simulink model "V2G_FDCC"  (R2024a)
settings: Solver=FixedStepAuto  StartTime=0.0  StopTime=20  FixedStep=1e-5  MaxStep=1.0E-5  RelTol=1e-3
values from neighbouring files (symbols this model uses):
  C_inv = (r*(Pinv/3)*al*(-be+al-1))/(100*Vac_l_rms*Vin_inv*wn*(al-be))    [main_v2gg2v.m]
  C_mppt = 20*(Iout_mppt*D_mppt)/(deltaV*fs_mppt)    (= 0.0948148148148)    [main_v2gg2v.m]
  cap_bat = 2000    [main_v2gg2v.m]
  Cbat_buck = deltaI_bat/(8*fs_bat*deltaV_bat)    (= 0.00133333333333)    [main_v2gg2v.m]
  Cdc = 30e-3    (= 0.03)    [main_v2gg2v.m]
  Cdc_boost = 50*Cbat_buck    (= 0.0666666666667)    [main_v2gg2v.m]
  D = 5    [main_v2gg2v.m]    (also in test.m = [0; 1; 4; 8; 1; 10; 0.5; 0.1; 0.5; 2; 4; 12; 1; 1; 1; 1])
  Dinv = results.Dinv(comb_idx)    [calculate_cct.m]    (also in main_v2gg2v.m = 7)
  f_grid = 50    [main_v2gg2v.m]
  fg = 50    [main_v2gg2v.m]
  H1 = 3    [main_v2gg2v.m]
  H2 = 4    [main_v2gg2v.m]
  H3 = 5    [main_v2gg2v.m]
  Hinv = results.Hinv(comb_idx)    [calculate_cct.m]    (also in main_v2gg2v.m = 3)
  L_bat = (Vbat*(Vdc_link-Vbat))/(deltaI_bat*fs_bat*Vdc_link)    (= 0.001875)    [main_v2gg2v.m]
  L_mppt = 1*(Vpv*D_mppt)/(deltaI*fs_mppt)    (= 0.000161333333333)    [main_v2gg2v.m]
  Lmin_inv = (100*Vac_l_rms*Vin_inv*(al-be))/(wn*r*(Pinv/3)*(-be+al-1))    [main_v2gg2v.m]
  Pinv = 2e6    (= 2000000)    [main_v2gg2v.m]
  Sbase = 1e6    (= 1000000)    [main_v2gg2v.m]
  t_fault_end = t_fault_start + FCT    [calculate_cct.m]    (also in main_v2gg2v.m = 1.02)
  t_fault_start = 1    [calculate_cct.m]    (also in main_v2gg2v.m)
  Vac_inv = 800    [main_v2gg2v.m]
  Vbase = 345e3    (= 345000)    [main_v2gg2v.m]
  Vbat = 750    [main_v2gg2v.m]
  wg = 2*pi*fg    (= 314.159265359)    [main_v2gg2v.m]
undefined symbols (not defined in the file or in its folder): Acid, D1, Delta, L12, L13, L23, Lead
libraries: spsGroundLib x48, spsSeriesRLCBranchLib x32, eeGeneralControl x27, slpidlib x24, spsCurrentMeasurementLib x18, spsThreePhaseSeriesRLCBranchLib x15, spsThreePhaseVIMeasurementLib x14, spsVoltageMeasurementLib x11, spsBatteryLib x10, spsMosfetLib x8, spsPWMGeneratorDCDCLib x8, spsabctodq0Lib x8
(part 1 of 4)
settings Model: SimulationMode=accelerator  Creator=BagaskaraPP  LastModifiedBy=hp
settings SolverCC: ZeroCrossAlgorithm=Adaptive  AlgebraicLoopSolver=TrustRegion
settings DataIOCC: ExternalInput=getinputstruct(op1)  InitialState=getstatestruct(op1)  SaveFinalState=on  SaveOperatingPoint=on  SaveFormat=Structure  ReturnWorkspaceOutputs=off  Refine=4
settings DebuggingCC: AlgebraicLoopMsg=none  MaxConsecutiveZCsMsg=none  IgnoredZcDiagnostic=none  ArithmeticOperatorsInVariantConditions=warning
settings ModelReferenceCC: EnableRefExpFcnMdlSchedulingChecks=on
settings SFSimCC: SimUseLocalCustomCode=off  CustomCodeUndefinedFunction=UseInterfaceOnly
settings RTWCC: RTWUseLocalCustomCode=off  GPUComputeCapability=3.5
settings CodeAppCC: StateflowObjectComments=on
settings SimscapeCC: SimscapeNormalizeSystem=off

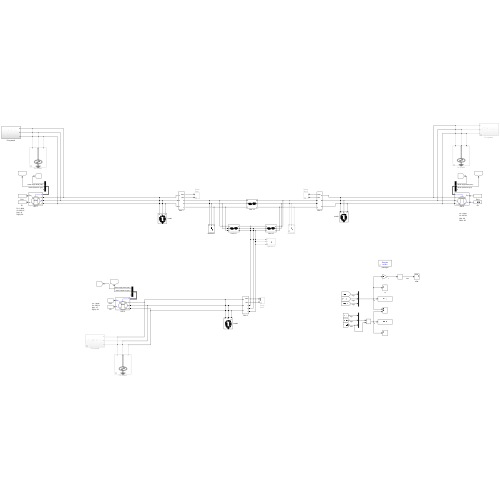
[thumbnail: Simulink's stored preview of the top-level diagram]
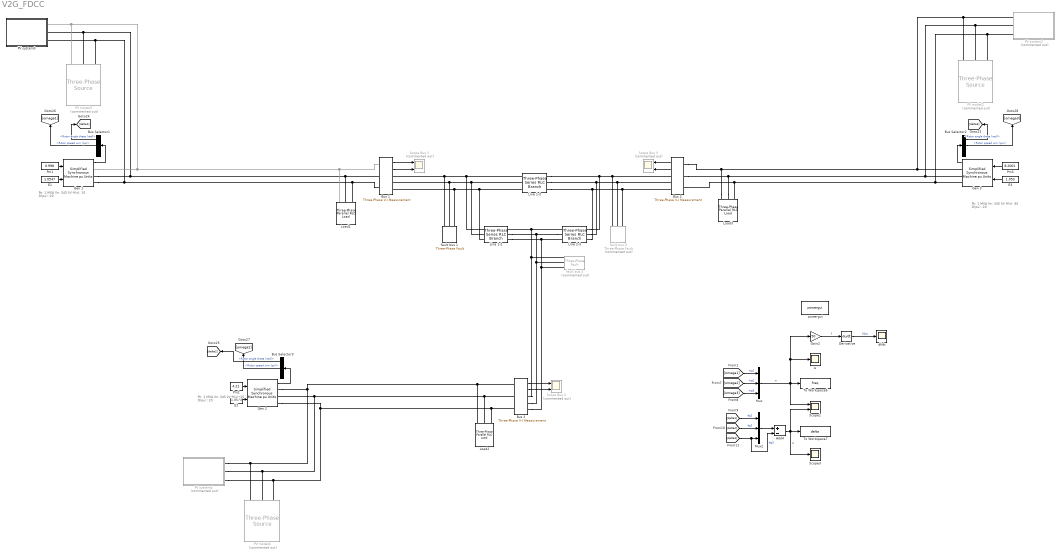
== system V2G_FDCC ==
  note: Pn: 1 MVA
      | Vn: 345 kV
      | H(s): 15
      | D(pu): 20
  note: Pn: 1 MVA
      | Vn: 345 kV
      | H(s): 60
      | D(pu): 20
  note: Pn: 1 MVA
      | Vn: 345 kV
      | H(s): 10
      | D(pu): 20
  Add4 : Sum  Inputs=+-
  Bus Selector1 : BusSelector  OutputSignals=Rotor angle theta (rad),Rotor speed wm (pu),Electrical power Pe (pu)
  Bus Selector2 : BusSelector  OutputSignals=Rotor angle theta (rad),Rotor speed wm (pu),Electrical power Pe (pu)
  Bus Selector3 : BusSelector  OutputSignals=Rotor angle theta (rad),Rotor speed wm (pu),Electrical power Pe (pu)
  Bus 1 : spsThreePhaseVIMeasurementLib/Three-Phase V-I Measurement  VoltageMeasurement=phase-to-ground  SetLabelV=off  LabelV=Vabc  Vpu=off  VpuLL=off  CurrentMeasurement=yes  SetLabelI=off  LabelI=Iabc  Ipu=off  Pbase=100e6  Vbase=500e3  OutputType=Complex  PhasorSimulation=off  PSBequivalent=0
  Bus 2 : spsThreePhaseVIMeasurementLib/Three-Phase V-I Measurement  VoltageMeasurement=phase-to-ground  SetLabelV=off  LabelV=Vabc  Vpu=off  VpuLL=off  CurrentMeasurement=yes  SetLabelI=off  LabelI=Iabc  Ipu=off  Pbase=100e6  Vbase=500e3  OutputType=Complex  PhasorSimulation=off  PSBequivalent=0
  Bus 3 : spsThreePhaseVIMeasurementLib/Three-Phase V-I Measurement  VoltageMeasurement=phase-to-ground  SetLabelV=off  LabelV=Vabc  Vpu=off  VpuLL=off  CurrentMeasurement=yes  SetLabelI=off  LabelI=Iabc  Ipu=off  Pbase=100e6  Vbase=500e3  OutputType=Complex  PhasorSimulation=off  PSBequivalent=0
  Derivative : Derivative
  E1 : Constant  Value=1.0547
  E2 : Constant  Value=1.0573
  E3 : Constant  Value=1.053
  Gain2 : Gain  Gain=50
  Gen 1 : spsSimplifiedSynchronousMachinepuUnitsLib/Simplified Synchronous Machine pu Units  ConnectionType=3-wire Y  MechanicalLoad=Mechanical power Pm  MeasurementBus=off  NominalParameters=[Sbase Vbase f_grid]  Mechanical=[H1 D 1]  InternalRL="[0.0  0.088]"  InitialConditions=[0 19.7182 1.15402 1.15402 1.15402 -15.1984 -135.198 104.802]  IterativeDiscreteModel=Trapezoidal non iterative  TsBlock=-1  TsPowergui=0  LoadFlowParameters=[1,0,0,0,0]  Units=0  BusType=PV  Pref=998000  Qref=0  Qmin=-Inf  Qmax=Inf  PLF=0  QLF=0
      settings: LibrarySourceBlock=|
      | sps_lib/Electrical Machines/Simplified Synchronous
      | Machine pu Units
  Gen 2 : spsSimplifiedSynchronousMachinepuUnitsLib/Simplified Synchronous Machine pu Units  ConnectionType=3-wire Y  MechanicalLoad=Mechanical power Pm  MeasurementBus=off  NominalParameters=[Sbase Vbase f_grid]  Mechanical=[H2 D 1]  InternalRL="[0.0  0.05]"  InitialConditions=[0 26.4702 4.27146 4.27146 4.27146 5.2548 -114.745 125.255]  IterativeDiscreteModel=Trapezoidal non iterative  TsBlock=-1  TsPowergui=0  LoadFlowParameters=[1,0,0,0,0]  Units=0  BusType=PV  Pref=4210000  Qref=0  Qmin=-Inf  Qmax=Inf  PLF=0  QLF=0
      settings: LibrarySourceBlock=|
      | sps_lib/Electrical Machines/Simplified Synchronous
      | Machine pu Units
  Gen 3 : spsSimplifiedSynchronousMachinepuUnitsLib/Simplified Synchronous Machine pu Units  ConnectionType=3-wire Y  MechanicalLoad=Mechanical power Pm  MeasurementBus=off  NominalParameters=[Sbase Vbase f_grid]  Mechanical=[H3 D 1]  InternalRL="[0.0  0.015]"  InitialConditions=[0 6.70815 8.74967 8.74967 8.74967 -20.4148 -140.415 99.5852]  IterativeDiscreteModel=Trapezoidal non iterative  TsBlock=-1  TsPowergui=0  LoadFlowParameters=[1,0,0,0,0]  Units=0  BusType=swing  Pref=6200000  Qref=0  Qmin=-Inf  Qmax=Inf  PLF=0  QLF=0
      settings: LibrarySourceBlock=|
      | sps_lib/Electrical Machines/Simplified Synchronous
      | Machine pu Units
  Line 1-2 : spsThreePhaseSeriesRLCBranchLib/Three-Phase Series RLC Branch  LConnTagsString=A|B|C  RConnTagsString=A|B|C  BranchType=RL  Resistance=0  Inductance=L12  Capacitance=1e-6  Measurements=None
  Line 1-3 : spsThreePhaseSeriesRLCBranchLib/Three-Phase Series RLC Branch  LConnTagsString=A|B|C  RConnTagsString=A|B|C  BranchType=RL  Resistance=0  Inductance=L13  Capacitance=1e-6  Measurements=None
  Line 2-3 : spsThreePhaseSeriesRLCBranchLib/Three-Phase Series RLC Branch  LConnTagsString=A|B|C  RConnTagsString=A|B|C  BranchType=RL  Resistance=0  Inductance=L23  Capacitance=1e-6  Measurements=None
  Load1 : spsThreePhaseParallelRLCLoadLib/Three-Phase Parallel RLC Load  LConnTagsString=A|B|C  Configuration=Y (grounded)  NominalVoltage=(345000)*1  Vabc=[1e3 1e3 1e3]  Vabcp=[1e3 1e3 1e3]  NominalFrequency=f_grid  UnbalancedPower=off  ActivePower=1500000  InductivePower=450000  CapacitivePower=0  Pabc=[10e3 9e3 11e3]  QLabc=[100 90 110]  QCabc=[100 90 110]  Pabcp=[10e3 9e3 11e3]  QLabcp=[100 90 110]  QCabcp=[100 90 110]  Measurements=None  LoadType=constant PQ
  Load2 : spsThreePhaseParallelRLCLoadLib/Three-Phase Parallel RLC Load  LConnTagsString=A|B|C  Configuration=Y (grounded)  NominalVoltage=(345000)*1  Vabc=[1e3 1e3 1e3]  Vabcp=[1e3 1e3 1e3]  NominalFrequency=f_grid  UnbalancedPower=off  ActivePower=1000000  InductivePower=300000  CapacitivePower=0  Pabc=[10e3 9e3 11e3]  QLabc=[100 90 110]  QCabc=[100 90 110]  Pabcp=[10e3 9e3 11e3]  QLabcp=[100 90 110]  QCabcp=[100 90 110]  Measurements=None  LoadType=constant PQ
  Load3 : spsThreePhaseParallelRLCLoadLib/Three-Phase Parallel RLC Load  LConnTagsString=A|B|C  Configuration=Y (grounded)  NominalVoltage=(345000)*1  Vabc=[1e3 1e3 1e3]  Vabcp=[1e3 1e3 1e3]  NominalFrequency=f_grid  UnbalancedPower=off  ActivePower=12400000  InductivePower=2500000  CapacitivePower=0  Pabc=[10e3 9e3 11e3]  QLabc=[100 90 110]  QCabc=[100 90 110]  Pabcp=[10e3 9e3 11e3]  QLabcp=[100 90 110]  QCabcp=[100 90 110]  Measurements=None  LoadType=constant PQ
  Mux : Mux  Inputs=3
  Mux1 : Mux  Inputs=3
  PV model2 : spsThreePhaseSourceLib/Three-Phase Source  Commented=on  InternalConnection=Yg  VoltagePhases=off  Voltage=(345000)*1  PhaseAngle=0  Voltage_phases=[25e3 25e3 25e3]/sqrt(3)  PhaseAngles_phases=[0 -120 +120]  Frequency=fg  NonIdealSource=off  SpecifyImpedance=off  Resistance=0.8929  Inductance=16.58e-3  ShortCircuitLevel=100e6  BaseVoltage=25e3  XRratio=7  BusType=PQ  Pref=1492000  Qref=606.9  Prefabc=[10e3, 10e3, 10e3]  Qrefabc=[0, 0, 0]  Qmin=-Inf  Qmax=Inf
  PV model3 : spsThreePhaseSourceLib/Three-Phase Source  Commented=on  InternalConnection=Yg  VoltagePhases=off  Voltage=(345000)*1  PhaseAngle=14.9415  Voltage_phases=[25e3 25e3 25e3]/sqrt(3)  PhaseAngles_phases=[0 -120 +120]  Frequency=fg  NonIdealSource=off  SpecifyImpedance=off  Resistance=0.8929  Inductance=16.58e-3  ShortCircuitLevel=100e6  BaseVoltage=25e3  XRratio=7  BusType=PQ  Pref=1492000  Qref=606.9  Prefabc=[10e3, 10e3, 10e3]  Qrefabc=[0, 0, 0]  Qmin=-Inf  Qmax=Inf
  PV model4 : spsThreePhaseSourceLib/Three-Phase Source  Commented=on  InternalConnection=Yg  VoltagePhases=off  Voltage=(345000)*1  PhaseAngle=21.4896  Voltage_phases=[25e3 25e3 25e3]/sqrt(3)  PhaseAngles_phases=[0 -120 +120]  Frequency=fg  NonIdealSource=off  SpecifyImpedance=off  Resistance=0.8929  Inductance=16.58e-3  ShortCircuitLevel=100e6  BaseVoltage=25e3  XRratio=7  BusType=PQ  Pref=1492000  Qref=606.9  Prefabc=[10e3, 10e3, 10e3]  Qrefabc=[0, 0, 0]  Qmin=-Inf  Qmax=Inf
  PV system2 : Subsystem  Commented=on
  PV system3 : Subsystem
  PV system4 : Subsystem  Commented=on
  Pm1 : Constant  Value=0.998
  Pm2 : Constant  Value=4.21
  Pm3 : Constant  Value=8.2001
  Scope Bus 1 : Scope  Commented=on  NumInputPorts=2
  Scope Bus 2 : Scope  Commented=on  NumInputPorts=2
  Scope Bus 3 : Scope  Commented=on  NumInputPorts=2
  Scope1 : Scope  NumInputPorts=2
  Scope3 : Scope
  To Workspace6 : ToWorkspace  VariableName=freq  SaveFormat=Timeseries  SampleTime=-1
  To Workspace7 : ToWorkspace  VariableName=delta  SaveFormat=Timeseries  SampleTime=-1
  df/dt : Scope
  fault bus 1 : spsThreePhaseFaultLib/Three-Phase Fault  InitialStates=0  FaultA=on  FaultB=on  FaultC=on  GroundFault=off  SwitchTimes="[t_fault_start  t_fault_end]"  External=off  SwitchStatus=NaN  FaultResistance=0.001  GroundResistance=0.01  SnubberResistance=inf  SnubberCapacitance=inf  Measurements=None
  fault bus 2 : spsThreePhaseFaultLib/Three-Phase Fault  Commented=on  InitialStates=0  FaultA=on  FaultB=on  FaultC=on  GroundFault=off  SwitchTimes="[t_fault_start  t_fault_end]"  External=off  SwitchStatus=NaN  FaultResistance=0.001  GroundResistance=0.01  SnubberResistance=inf  SnubberCapacitance=inf  Measurements=None
  fault bus 3 : spsThreePhaseFaultLib/Three-Phase Fault  Commented=on  InitialStates=0  FaultA=on  FaultB=on  FaultC=on  GroundFault=off  SwitchTimes="[t_fault_start  t_fault_end]"  External=off  SwitchStatus=NaN  FaultResistance=0.001  GroundResistance=0.01  SnubberResistance=inf  SnubberCapacitance=inf  Measurements=None
  powergui : sps_lib/powergui  Priority=1  SimulationMode=Discrete  SampleTime=1e-5  frequency=60  Iterations=200  frequencyindice=50  Pbase=1e6  ErrMax=1e-4  UnitsV=kV  UnitsW=MW  buscounter=1  FunctionMessages=off  echomessages=off  EnableUseOfTLC=off  CurrentSourceSwitches=off  DisableSnubberDevices=off  DisableRonSwitches=off  DisableVfSwitches=off  DisplayEquations=off  AutomaticDiscreteSolvers=off  SolverType=Tustin/Backward Euler (TBE)  Interpol=off  ExternalGateDelay=off  methode=off  Ts=100  x0status=blocks  SPID=on  SwTol=0  HookPort=off  NonlinearTolerance=1e-4  nMaxIteration=100  ContinueOnMaxIteration=off  RestoreLinks=warning  ResistiveCurrentMeasurement=off  Frange=[0:2:500]  Ylog=off  Xlog=on  ShowGrid=off  save=off  variable=ZData  structure=0  ZoomFFT=off  StartTime=0.0  cycles=1  DisplayStyle=1  fundamental=60  FreqAxis=off  MaxFrequency=1000  frequencyindicesteady=1  RmsSteady=1  display=off
  w : Scope
  wires:
  Bus 1/1 -> Scope Bus 1/1
  Pm2/1 -> Gen 2/1
  Bus Selector2/2 -> [omega3]  "<Rotor speed wm (pu)>"
  Bus Selector2/1 -> [delta3]  "<Rotor angle theta (rad)>"
  Pm3/1 -> Gen 3/1
  Bus 2/2 -> Scope Bus 2/2
  Bus 1/2 -> Scope Bus 1/2
  Bus Selector3/2 -> [omega2]  "<Rotor speed wm (pu)>"
  Bus 3/2 -> Scope Bus 3/2
  Bus Selector3/1 -> [delta2]  "<Rotor angle theta (rad)>"
  Bus 3/1 -> Scope Bus 3/1
  Bus 2/1 -> Scope Bus 2/1
  E1/1 -> Gen 1/2
  Pm1/1 -> Gen 1/1
  Gen 1/1 -> Bus Selector1/1
  Gen 3/1 -> Bus Selector2/1
  Bus Selector1/2 -> [omega1]  "<Rotor speed wm (pu)>"
  Bus Selector1/1 -> [delta1]  "<Rotor angle theta (rad)>"
  Gen 2/1 -> Bus Selector3/1
  E2/1 -> Gen 2/2
  E3/1 -> Gen 3/2
  Mux/1 -> Scope1/1, Gain2/1, w/1, To Workspace6/1  "w"
  Gain2/1 -> Derivative/1  "f"
  [delta3] -> Add4/2, Mux1/3  "dg3"
  Derivative/1 -> df/dt/1  "fdot"
  Add4/1 -> Scope1/2, Scope3/1, To Workspace7/1  "d"
  Mux1/1 -> Add4/1
  [delta1] -> Mux1/1  "dg1"
  [delta2] -> Mux1/2  "dg2"
  [omega2] -> Mux/2  "wg2"
  [omega1] -> Mux/1  "wg1"
  [omega3] -> Mux/3  "wg3"
  connections:
  Line 1-2/LConn1 -- Line 1-3/LConn1 -- fault bus 1/LConn1 -- Bus 1/RConn1
  Load1/LConn3 -- PV system3/RConn3 -- PV model3/RConn3 -- Gen 1/RConn3 -- Bus 1/LConn3
  Line 2-3/LConn2 -- Bus 2/RConn2 -- fault bus 2/LConn2 -- Line 1-2/RConn2
  Gen 3/RConn3 -- Bus 3/LConn3 -- Load3/LConn3 -- PV model2/RConn3 -- PV system2/RConn3
  Bus 3/RConn2 -- fault bus 3/LConn2 -- Line 2-3/RConn2 -- Line 1-3/RConn2
  Bus 3/RConn3 -- fault bus 3/LConn3 -- Line 2-3/RConn3 -- Line 1-3/RConn3
  PV system3/RConn2 -- PV model3/RConn2 -- Load1/LConn2 -- Bus 1/LConn2 -- Gen 1/RConn2
  Load3/LConn1 -- PV model2/RConn1 -- PV system2/RConn1 -- Gen 3/RConn1 -- Bus 3/LConn1
  Line 2-3/LConn1 -- Bus 2/RConn1 -- fault bus 2/LConn1 -- Line 1-2/RConn1
  Load3/LConn2 -- PV model2/RConn2 -- PV system2/RConn2 -- Gen 3/RConn2 -- Bus 3/LConn2
  Line 1-3/RConn1 -- Bus 3/RConn1 -- fault bus 3/LConn1 -- Line 2-3/RConn1
  Line 1-3/LConn2 -- Line 1-2/LConn2 -- fault bus 1/LConn2 -- Bus 1/RConn2
  Line 1-2/LConn3 -- Line 1-3/LConn3 -- fault bus 1/LConn3 -- Bus 1/RConn3
  PV model3/RConn1 -- PV system3/RConn1 -- Load1/LConn1 -- Bus 1/LConn1 -- Gen 1/RConn1
  Bus 2/RConn3 -- fault bus 2/LConn3 -- Line 2-3/LConn3 -- Line 1-2/RConn3
  Gen 2/RConn1 -- Load2/LConn1 -- Bus 2/LConn1 -- PV model4/RConn1 -- PV system4/RConn1
  Load2/LConn2 -- PV model4/RConn2 -- PV system4/RConn2 -- Gen 2/RConn2 -- Bus 2/LConn2
  Gen 2/RConn3 -- PV model4/RConn3 -- PV system4/RConn3 -- Bus 2/LConn3 -- Load2/LConn3

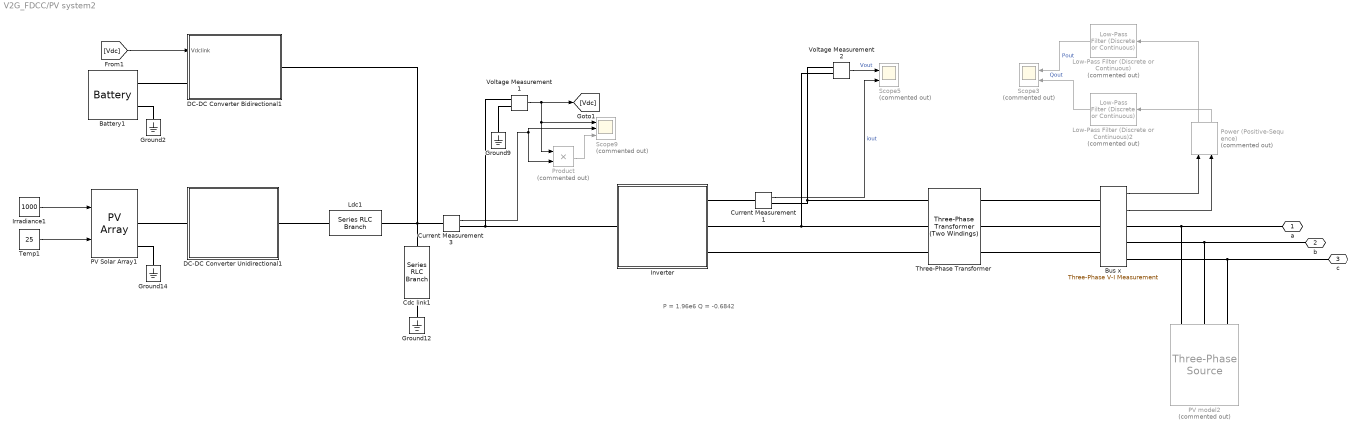
== system V2G_FDCC/PV system2 ==
  note: P = 1.96e6
      | Q = -0.6842
  Battery1 : spsBatteryLib/Battery  BatType=Lead-Acid  ShowTempParam=off  ThermalPreset="12.8V  40Ah  (LiFeMgPO4)"  ShowAgeParam=off  NomV=Vbat  NomQ=cap_bat  SOC=50  Batt_Tr=2  PresetModel=off  MaxQ=cap_bat  MinV=0.8*Vbat  FullV=1.1*Vbat  Dis_rate=Inom_bat  R=0.002  Normal_OP=0.9*cap_bat  expZone="[780   20]"  current=[250 500 750 1000]  Units=Ampere-hour  Tci=20  NomT=20  T2=-30  MaxQ2=4.8  FullV2=7.1  Normal_OP2=5.655  expZone2="[6.58           1]"  Rca=0.6  ti=2000  Dp=0  Neq0=0  Tsim=1e6  Ta1=25  Qeol=5.4*0.9  Reol=0.013333*1.2  Char_age=[2.3478, 3]  Dis_age=[2.3478, 10]  N1=1500  N2=10500  N3=1000  N4=1400  Ta2=45  N5=950
  Bus x : spsThreePhaseVIMeasurementLib/Three-Phase V-I Measurement  VoltageMeasurement=phase-to-ground  SetLabelV=off  LabelV=Vabc  Vpu=off  VpuLL=off  CurrentMeasurement=yes  SetLabelI=off  LabelI=Iabc  Ipu=off  Pbase=100e6  Vbase=13.8e3  OutputType=Complex  PhasorSimulation=off  PSBequivalent=0
  Cdc link1 : spsSeriesRLCBranchLib/Series RLC Branch  LConnTagsString=__new0  RConnTagsString=__new0  BranchType=C  Resistance=0.001  Inductance=1e-3  SetiL0=off  InitialCurrent=0  Capacitance=Cdc  Setx0=on  InitialVoltage=1500  Measurements=None
  Current Measurement1 : spsCurrentMeasurementLib/Current Measurement  PhasorSimulation=off  OutputType=Complex  PSBequivalent=0
  Current Measurement3 : spsCurrentMeasurementLib/Current Measurement  PhasorSimulation=off  OutputType=Complex  PSBequivalent=0
  DC-DC Converter Bidirectional1 : Subsystem
  DC-DC Converter Unidirectional1 : Subsystem
  Ground{2,9,12,14} (4 alike) : spsGroundLib/Ground  LConnTagsString=a
  Inverter : Subsystem
  Irradiance1 : Constant  Value=1000
  Ldc1 : spsSeriesRLCBranchLib/Series RLC Branch  LConnTagsString=__new0  RConnTagsString=__new0  BranchType=L  Resistance=0.002  Inductance=10e-3  SetiL0=off  InitialCurrent=0  Capacitance=5e-3  Setx0=on  InitialVoltage=0  Measurements=None
  Low-Pass Filter (Discrete or Continuous) : eeGeneralControl/Low-Pass Filter (Discrete or Continuous)  Commented=on  K=1  T=1/(2*pi*5)  B=inf  A=-inf  init_option=Inherited from block input  x0=0  Ts=-1
  Low-Pass Filter (Discrete or Continuous)2 : eeGeneralControl/Low-Pass Filter (Discrete or Continuous)  Commented=on  K=1  T=1/(2*pi*5)  B=inf  A=-inf  init_option=Inherited from block input  x0=0  Ts=-1
  PV Solar Array1 : spsPVArrayLib/PV Array  Npar=278  Nser=15  PlotType=array @ 1000 W/m2 & specified temperatures  S_vec=[ 1000 800 500 300 100 ]  Temp_C_vec=[ 20 25 30 35 ]  ModuleName=Sunpower SPR-X22-480-COM  PlotWhenSelected=off  Pm=480.32  Ncell=128  Voc=92.9  Isc=6.48  Vm=79  Im=6.08  beta_Voc_pc=-0.293  alpha_Isc_pc=0.031003  beta_Voc=-0.2722  alpha_Isc=0.002009  IL=6.4884  I0=1.5908e-11  nI=1.0576  Rsh=598.2816  Rs=0.48607  RobustModel=off  RobustCellTemperature=313.3991  BAL=on  Tc=1e-6  Tfilter=5e-5
  PV model2 : spsThreePhaseSourceLib/Three-Phase Source  Commented=on  InternalConnection=Yg  VoltagePhases=off  Voltage=(345000)*1  PhaseAngle=0  Voltage_phases=[25e3 25e3 25e3]/sqrt(3)  PhaseAngles_phases=[0 -120 +120]  Frequency=fg  NonIdealSource=off  SpecifyImpedance=off  Resistance=0.8929  Inductance=16.58e-3  ShortCircuitLevel=100e6  BaseVoltage=25e3  XRratio=7  BusType=swing  Pref=1993000  Qref=10680  Prefabc=[10e3, 10e3, 10e3]  Qrefabc=[0, 0, 0]  Qmin=-Inf  Qmax=Inf
  Power (Positive-Sequence) : spsPowerPositiveSequenceLib/Power (Positive-Sequence)  Commented=on  Freq=50  Vinit=[0, 0]  Iinit=[0, 0]  Ts=1e-5
      settings: LibrarySourceBlock=|
      | sps_lib/Sensors and Measurements/Power
      | (Positive-Sequence)
  Product : Product  Commented=on
  Scope3 : Scope  Commented=on  NumInputPorts=2
  Scope5 : Scope  Commented=on  NumInputPorts=2
  Scope9 : Scope  Commented=on  NumInputPorts=3
  Temp1 : Constant  Value=25
  Three-Phase Transformer : spsThreePhaseTransformerTwoWindingsLib/Three-Phase Transformer (Two Windings)  Winding1Connection=Yg  Winding2Connection=Delta (D1)  CoreType=Three single-phase transformers  SetSaturation=off  Hysteresis=off  DataFile='hysteresis'  SetInitialFlux=off  Measurements=None  UNITS=pu  NominalPower=[ Pinv*2 , fg ]  Winding1=[Vbase 1e-6 1e-6]  Winding2=[Vac_inv 1e-6 1e-6]  Rm=500  Lm=1000  L0=0.5  Saturation=[0 0;0.01 0.9;0.05 1]  InitialFluxes=[-1.0025142026259 0.501432695325379 0.501081507300505]  BreakLoop=off  DiscreteSolver=Trapezoidal iterative  DataType=off  TransfoNumber=1
  Voltage Measurement1 : spsVoltageMeasurementLib/Voltage Measurement  PhasorSimulation=off  OutputType=Complex  PSBequivalent=0
  Voltage Measurement2 : spsVoltageMeasurementLib/Voltage Measurement  PhasorSimulation=off  OutputType=Complex  PSBequivalent=0
  a : PMIOPort  Side=Right
  b : PMIOPort  Port=2  Side=Right
  c : PMIOPort  Port=3  Side=Right
  wires:
  Voltage Measurement2/1 -> Scope5/1  "Vout"
  Irradiance1/1 -> PV Solar Array1/1
  Low-Pass Filter (Discrete or Continuous)/1 -> Scope3/1  "Pout"
  Power (Positive-Sequence)/1 -> Low-Pass Filter (Discrete or Continuous)/1
  Current Measurement1/1 -> Scope5/2  "iout"
  Voltage Measurement1/1 -> [Vdc], Product/1, Scope9/1
  Current Measurement3/1 -> Product/2, Scope9/2
  Low-Pass Filter (Discrete or Continuous)2/1 -> Scope3/2  "Qout"
  [Vdc] -> DC-DC Converter Bidirectional1/1(Vdclink)
  Bus x/2 -> Power (Positive-Sequence)/2
  Temp1/1 -> PV Solar Array1/2
  Bus x/1 -> Power (Positive-Sequence)/1
  Power (Positive-Sequence)/2 -> Low-Pass Filter (Discrete or Continuous)2/1
  Product/1 -> Scope9/3
  connections:
  Inverter/RConn1 -- Current Measurement1/LConn1
  PV Solar Array1/RConn1 -- DC-DC Converter Unidirectional1/LConn1
  Voltage Measurement2/LConn1 -- Current Measurement1/RConn1 -- Three-Phase Transformer/RConn1
  Voltage Measurement2/LConn2 -- Inverter/RConn2 -- Three-Phase Transformer/RConn2
  Inverter/LConn1 -- Voltage Measurement1/LConn1 -- Current Measurement3/RConn1
  Three-Phase Transformer/RConn3 -- Inverter/RConn3
  Battery1/LConn2 -- Ground2/LConn1
  Three-Phase Transformer/LConn3 -- Bus x/LConn3
  Voltage Measurement1/LConn2 -- Ground9/LConn1
  PV Solar Array1/RConn2 -- Ground14/LConn1
  Battery1/LConn1 -- DC-DC Converter Bidirectional1/LConn1
  Ground12/LConn1 -- Cdc link1/RConn1
  Three-Phase Transformer/LConn1 -- Bus x/LConn1
  Current Measurement3/LConn1 -- Cdc link1/LConn1 -- DC-DC Converter Bidirectional1/RConn1 -- Ldc1/RConn1
  Three-Phase Transformer/LConn2 -- Bus x/LConn2
  Ldc1/LConn1 -- DC-DC Converter Unidirectional1/RConn1
  Bus x/RConn2 -- b/RConn1 -- PV model2/RConn2
  Bus x/RConn1 -- a/RConn1 -- PV model2/RConn1
  Bus x/RConn3 -- c/RConn1 -- PV model2/RConn3

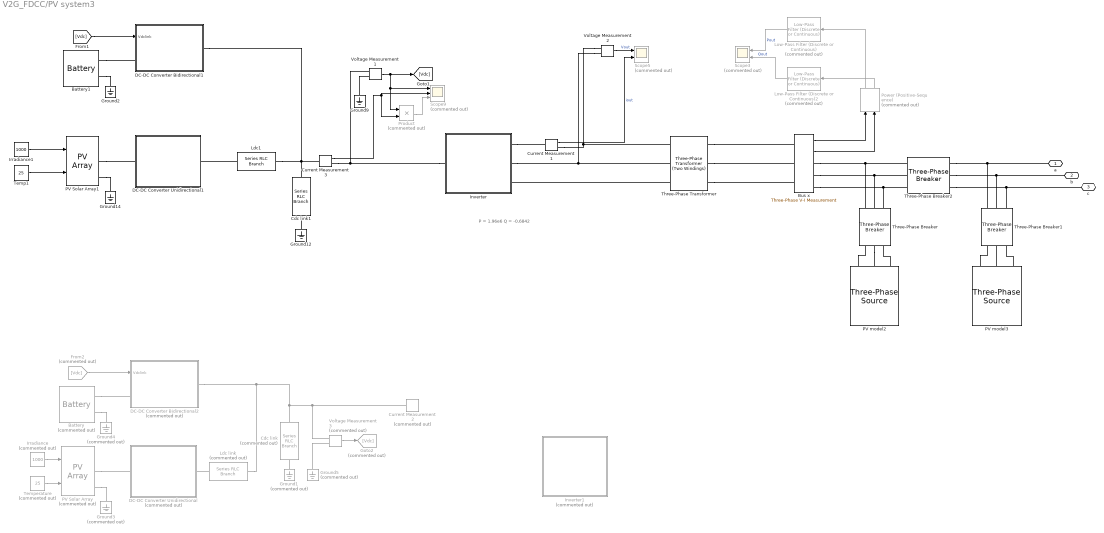
== system V2G_FDCC/PV system3 ==
  note: P = 1.96e6
      | Q = -0.6842
  Battery : spsBatteryLib/Battery  Commented=on  BatType=Lead-Acid  ShowTempParam=off  ThermalPreset="12.8V  40Ah  (LiFeMgPO4)"  ShowAgeParam=off  NomV=Vbat  NomQ=cap_bat  SOC=50  Batt_Tr=2  PresetModel=off  MaxQ=cap_bat  MinV=0.8*Vbat  FullV=1.1*Vbat  Dis_rate=Inom_bat  R=0.002  Normal_OP=0.9*cap_bat  expZone="[780   20]"  current=[250 500 750 1000]  Units=Ampere-hour  Tci=20  NomT=20  T2=-30  MaxQ2=4.8  FullV2=7.1  Normal_OP2=5.655  expZone2="[6.58           1]"  Rca=0.6  ti=2000  Dp=0  Neq0=0  Tsim=1e6  Ta1=25  Qeol=5.4*0.9  Reol=0.013333*1.2  Char_age=[2.3478, 3]  Dis_age=[2.3478, 10]  N1=1500  N2=10500  N3=1000  N4=1400  Ta2=45  N5=950
  Battery1 : spsBatteryLib/Battery  BatType=Lead-Acid  ShowTempParam=off  ThermalPreset="12.8V  40Ah  (LiFeMgPO4)"  ShowAgeParam=off  NomV=Vbat  NomQ=cap_bat  SOC=50  Batt_Tr=2  PresetModel=off  MaxQ=cap_bat  MinV=0.8*Vbat  FullV=1.1*Vbat  Dis_rate=Inom_bat  R=0.002  Normal_OP=0.9*cap_bat  expZone="[780   20]"  current=[250 500 750 1000]  Units=Ampere-hour  Tci=20  NomT=20  T2=-30  MaxQ2=4.8  FullV2=7.1  Normal_OP2=5.655  expZone2="[6.58           1]"  Rca=0.6  ti=2000  Dp=0  Neq0=0  Tsim=1e6  Ta1=25  Qeol=5.4*0.9  Reol=0.013333*1.2  Char_age=[2.3478, 3]  Dis_age=[2.3478, 10]  N1=1500  N2=10500  N3=1000  N4=1400  Ta2=45  N5=950
      link override Model/Exp/Discrete-Time Integrator: InitialCondition=7.56607358162621
  Bus x : spsThreePhaseVIMeasurementLib/Three-Phase V-I Measurement  VoltageMeasurement=phase-to-ground  SetLabelV=off  LabelV=Vabc  Vpu=off  VpuLL=off  CurrentMeasurement=yes  SetLabelI=off  LabelI=Iabc  Ipu=off  Pbase=100e6  Vbase=13.8e3  OutputType=Complex  PhasorSimulation=off  PSBequivalent=0
  Cdc link : spsSeriesRLCBranchLib/Series RLC Branch  Commented=on  LConnTagsString=__new0  RConnTagsString=__new0  BranchType=C  Resistance=0.001  Inductance=1e-3  SetiL0=off  InitialCurrent=0  Capacitance=Cdc  Setx0=on  InitialVoltage=1500  Measurements=None
  Cdc link1 : spsSeriesRLCBranchLib/Series RLC Branch  LConnTagsString=__new0  RConnTagsString=__new0  BranchType=C  Resistance=0.001  Inductance=1e-3  SetiL0=off  InitialCurrent=0  Capacitance=Cdc  Setx0=on  InitialVoltage=1500  Measurements=None
  Current Measurement1 : spsCurrentMeasurementLib/Current Measurement  PhasorSimulation=off  OutputType=Complex  PSBequivalent=0
  Current Measurement2 : spsCurrentMeasurementLib/Current Measurement  Commented=on  PhasorSimulation=off  OutputType=Complex  PSBequivalent=0
  Current Measurement3 : spsCurrentMeasurementLib/Current Measurement  PhasorSimulation=off  OutputType=Complex  PSBequivalent=0
  DC-DC Converter Bidirectional1 : Subsystem
  DC-DC Converter Bidirectional2 : Subsystem  Commented=on
  DC-DC Converter Unidirectional : Subsystem  Commented=on
  DC-DC Converter Unidirectional1 : Subsystem
  From2 : From  Commented=on  GotoTag=Vdc
  Goto2 : Goto  Commented=on  GotoTag=Vdc
  Ground{1,3..5} (4 alike) : spsGroundLib/Ground  Commented=on  LConnTagsString=a
  Ground{2,9,12,14} (4 alike) : spsGroundLib/Ground  LConnTagsString=a
  Inverter : Subsystem
  Inverter1 : Subsystem  Commented=on
  Irradiance : Constant  Commented=on  Value=1000
  Irradiance1 : Constant  Value=1000
  Ldc link : spsSeriesRLCBranchLib/Series RLC Branch  Commented=on  LConnTagsString=__new0  RConnTagsString=__new0  BranchType=L  Resistance=0.002  Inductance=10e-3  SetiL0=off  InitialCurrent=0  Capacitance=5e-3  Setx0=on  InitialVoltage=0  Measurements=None
  Ldc1 : spsSeriesRLCBranchLib/Series RLC Branch  LConnTagsString=__new0  RConnTagsString=__new0  BranchType=L  Resistance=0.002  Inductance=10e-3  SetiL0=off  InitialCurrent=0  Capacitance=5e-3  Setx0=on  InitialVoltage=0  Measurements=None
  Low-Pass Filter (Discrete or Continuous) : eeGeneralControl/Low-Pass Filter (Discrete or Continuous)  Commented=on  K=1  T=1/(2*pi*5)  B=inf  A=-inf  init_option=Inherited from block input  x0=0  Ts=-1
  Low-Pass Filter (Discrete or Continuous)2 : eeGeneralControl/Low-Pass Filter (Discrete or Continuous)  Commented=on  K=1  T=1/(2*pi*5)  B=inf  A=-inf  init_option=Inherited from block input  x0=0  Ts=-1
  PV Solar Array : spsPVArrayLib/PV Array  Commented=on  Npar=278  Nser=15  PlotType=array @ 1000 W/m2 & specified temperatures  S_vec=[ 1000 800 500 300 100 ]  Temp_C_vec=[ 20 25 30 35 ]  ModuleName=Sunpower SPR-X22-480-COM  PlotWhenSelected=off  Pm=480.32  Ncell=128  Voc=92.9  Isc=6.48  Vm=79  Im=6.08  beta_Voc_pc=-0.293  alpha_Isc_pc=0.031003  beta_Voc=-0.2722  alpha_Isc=0.002009  IL=6.4884  I0=1.5908e-11  nI=1.0576  Rsh=598.2816  Rs=0.48607  RobustModel=off  RobustCellTemperature=313.3991  BAL=on  Tc=1e-6  Tfilter=5e-5
  PV Solar Array1 : spsPVArrayLib/PV Array  Npar=278  Nser=15  PlotType=array @ 1000 W/m2 & specified temperatures  S_vec=[ 1000 800 500 300 100 ]  Temp_C_vec=[ 20 25 30 35 ]  ModuleName=Sunpower SPR-X22-480-COM  PlotWhenSelected=off  Pm=480.32  Ncell=128  Voc=92.9  Isc=6.48  Vm=79  Im=6.08  beta_Voc_pc=-0.293  alpha_Isc_pc=0.031003  beta_Voc=-0.2722  alpha_Isc=0.002009  IL=6.4884  I0=1.5908e-11  nI=1.0576  Rsh=598.2816  Rs=0.48607  RobustModel=off  RobustCellTemperature=313.3991  BAL=on  Tc=1e-6  Tfilter=5e-5
      link override Diode Rsh/Unit Delay: InitialCondition=56.2557232679295
  PV model2 : spsThreePhaseSourceLib/Three-Phase Source  InternalConnection=Yg  VoltagePhases=off  Voltage=(345000)*1  PhaseAngle=0  Voltage_phases=[25e3 25e3 25e3]/sqrt(3)  PhaseAngles_phases=[0 -120 +120]  Frequency=fg  NonIdealSource=off  SpecifyImpedance=off  Resistance=0.8929  Inductance=16.58e-3  ShortCircuitLevel=100e6  BaseVoltage=25e3  XRratio=7  BusType=swing  Pref=1993000  Qref=10680  Prefabc=[10e3, 10e3, 10e3]  Qrefabc=[0, 0, 0]  Qmin=-Inf  Qmax=Inf
  PV model3 : spsThreePhaseSourceLib/Three-Phase Source  InternalConnection=Yg  VoltagePhases=off  Voltage=(345000)*1  PhaseAngle=14.9415  Voltage_phases=[25e3 25e3 25e3]/sqrt(3)  PhaseAngles_phases=[0 -120 +120]  Frequency=fg  NonIdealSource=off  SpecifyImpedance=off  Resistance=0.8929  Inductance=16.58e-3  ShortCircuitLevel=100e6  BaseVoltage=25e3  XRratio=7  BusType=PQ  Pref=1492000  Qref=606.9  Prefabc=[10e3, 10e3, 10e3]  Qrefabc=[0, 0, 0]  Qmin=-Inf  Qmax=Inf
  Power (Positive-Sequence) : spsPowerPositiveSequenceLib/Power (Positive-Sequence)  Commented=on  Freq=50  Vinit=[0, 0]  Iinit=[0, 0]  Ts=1e-5
      settings: LibrarySourceBlock=|
      | sps_lib/Sensors and Measurements/Power
      | (Positive-Sequence)
  Product : Product  Commented=on
  Scope3 : Scope  Commented=on  NumInputPorts=2
  Scope5 : Scope  Commented=on  NumInputPorts=2
  Scope9 : Scope  Commented=on  NumInputPorts=3
  Temp1 : Constant  Value=25
  Temperature : Constant  Commented=on  Value=25
  Three-Phase Transformer : spsThreePhaseTransformerTwoWindingsLib/Three-Phase Transformer (Two Windings)  Winding1Connection=Yg  Winding2Connection=Delta (D1)  CoreType=Three single-phase transformers  SetSaturation=off  Hysteresis=off  DataFile='hysteresis'  SetInitialFlux=off  Measurements=None  UNITS=pu  NominalPower=[ Pinv*2 , fg ]  Winding1=[Vbase 1e-6 1e-6]  Winding2=[Vac_inv 1e-6 1e-6]  Rm=500  Lm=1000  L0=0.5  Saturation=[0 0;0.01 0.9;0.05 1]  InitialFluxes=[-1.0025142026259 0.501432695325379 0.501081507300505]  BreakLoop=off  DiscreteSolver=Trapezoidal iterative  DataType=off  TransfoNumber=1
  Three-Phase Breaker : spsThreePhaseBreakerLib/Three-Phase Breaker  InitialState=closed  SwitchA=on  SwitchB=on  SwitchC=on  SwitchTimes=[0.5]  External=off  BreakerResistance=1e-6  SnubberResistance=1e12  SnubberCapacitance=1e-12  Measurements=None
  Three-Phase Breaker1 : spsThreePhaseBreakerLib/Three-Phase Breaker  InitialState=closed  SwitchA=on  SwitchB=on  SwitchC=on  SwitchTimes=[0.5]  External=off  BreakerResistance=1e-6  SnubberResistance=1e12  SnubberCapacitance=1e-12  Measurements=None
  Three-Phase Breaker2 : spsThreePhaseBreakerLib/Three-Phase Breaker  InitialState=open  SwitchA=on  SwitchB=on  SwitchC=on  SwitchTimes=[0.5]  External=off  BreakerResistance=1e-6  SnubberResistance=1e12  SnubberCapacitance=1e-12  Measurements=None
  Voltage Measurement1 : spsVoltageMeasurementLib/Voltage Measurement  PhasorSimulation=off  OutputType=Complex  PSBequivalent=0
  Voltage Measurement2 : spsVoltageMeasurementLib/Voltage Measurement  PhasorSimulation=off  OutputType=Complex  PSBequivalent=0
  Voltage Measurement3 : spsVoltageMeasurementLib/Voltage Measurement  Commented=on  PhasorSimulation=off  OutputType=Complex  PSBequivalent=0
  a : PMIOPort  Side=Right
  b : PMIOPort  Port=2  Side=Right
  c : PMIOPort  Port=3  Side=Right
  wires:
  Voltage Measurement2/1 -> Scope5/1  "Vout"
  Irradiance1/1 -> PV Solar Array1/1
  Low-Pass Filter (Discrete or Continuous)/1 -> Scope3/1  "Pout"
  Power (Positive-Sequence)/1 -> Low-Pass Filter (Discrete or Continuous)/1
  Current Measurement1/1 -> Scope5/2  "iout"
  Voltage Measurement1/1 -> [Vdc], Product/1, Scope9/1
  Current Measurement3/1 -> Product/2, Scope9/2
  Low-Pass Filter (Discrete or Continuous)2/1 -> Scope3/2  "Qout"
  [Vdc] -> DC-DC Converter Bidirectional1/1(Vdclink)
  Bus x/2 -> Power (Positive-Sequence)/2
  Temp1/1 -> PV Solar Array1/2
  Bus x/1 -> Power (Positive-Sequence)/1
  Power (Positive-Sequence)/2 -> Low-Pass Filter (Discrete or Continuous)2/1
  Product/1 -> Scope9/3
  Temperature/1 -> PV Solar Array/2
  Voltage Measurement3/1 -> Goto2/1
  From2/1 -> DC-DC Converter Bidirectional2/1(Vdclink)
  Irradiance/1 -> PV Solar Array/1
  connections:
  Inverter/RConn1 -- Current Measurement1/LConn1
  PV Solar Array1/RConn1 -- DC-DC Converter Unidirectional1/LConn1
  Voltage Measurement2/LConn1 -- Current Measurement1/RConn1 -- Three-Phase Transformer/RConn1
  Voltage Measurement2/LConn2 -- Inverter/RConn2 -- Three-Phase Transformer/RConn2
  Inverter/LConn1 -- Voltage Measurement1/LConn1 -- Current Measurement3/RConn1
  Three-Phase Transformer/RConn3 -- Inverter/RConn3
  Battery1/LConn2 -- Ground2/LConn1
  Three-Phase Transformer/LConn3 -- Bus x/LConn3
  Voltage Measurement1/LConn2 -- Ground9/LConn1
  PV Solar Array1/RConn2 -- Ground14/LConn1
  Battery1/LConn1 -- DC-DC Converter Bidirectional1/LConn1
  Ground12/LConn1 -- Cdc link1/RConn1
  Three-Phase Transformer/LConn1 -- Bus x/LConn1
  Current Measurement3/LConn1 -- Cdc link1/LConn1 -- DC-DC Converter Bidirectional1/RConn1 -- Ldc1/RConn1
  Three-Phase Transformer/LConn2 -- Bus x/LConn2
  Ldc1/LConn1 -- DC-DC Converter Unidirectional1/RConn1
  Three-Phase Breaker/LConn2 -- PV model2/RConn2
  Bus x/RConn1 -- Three-Phase Breaker/RConn1 -- Three-Phase Breaker2/LConn1
  Ldc link/RConn1 -- Cdc link/LConn1 -- Current Measurement2/LConn1 -- Voltage Measurement3/LConn1 -- DC-DC Converter Bidirectional2/RConn1
  Ldc link/LConn1 -- DC-DC Converter Unidirectional/RConn1
  PV Solar Array/RConn1 -- DC-DC Converter Unidirectional/LConn1
  PV Solar Array/RConn2 -- Ground3/LConn1
  Voltage Measurement3/LConn2 -- Ground5/LConn1
  Ground1/LConn1 -- Cdc link/RConn1
  Battery/LConn2 -- Ground4/LConn1
  Battery/LConn1 -- DC-DC Converter Bidirectional2/LConn1
  PV model3/RConn1 -- Three-Phase Breaker1/LConn1
  PV model3/RConn2 -- Three-Phase Breaker1/LConn2
  PV model3/RConn3 -- Three-Phase Breaker1/LConn3
  Three-Phase Breaker2/RConn1 -- a/RConn1 -- Three-Phase Breaker1/RConn1
  Three-Phase Breaker2/RConn2 -- b/RConn1 -- Three-Phase Breaker1/RConn2
  Three-Phase Breaker2/RConn3 -- c/RConn1 -- Three-Phase Breaker1/RConn3
  Three-Phase Breaker2/LConn2 -- Bus x/RConn2 -- Three-Phase Breaker/RConn2
  Three-Phase Breaker2/LConn3 -- Bus x/RConn3 -- Three-Phase Breaker/RConn3
  PV model2/RConn1 -- Three-Phase Breaker/LConn1
  PV model2/RConn3 -- Three-Phase Breaker/LConn3

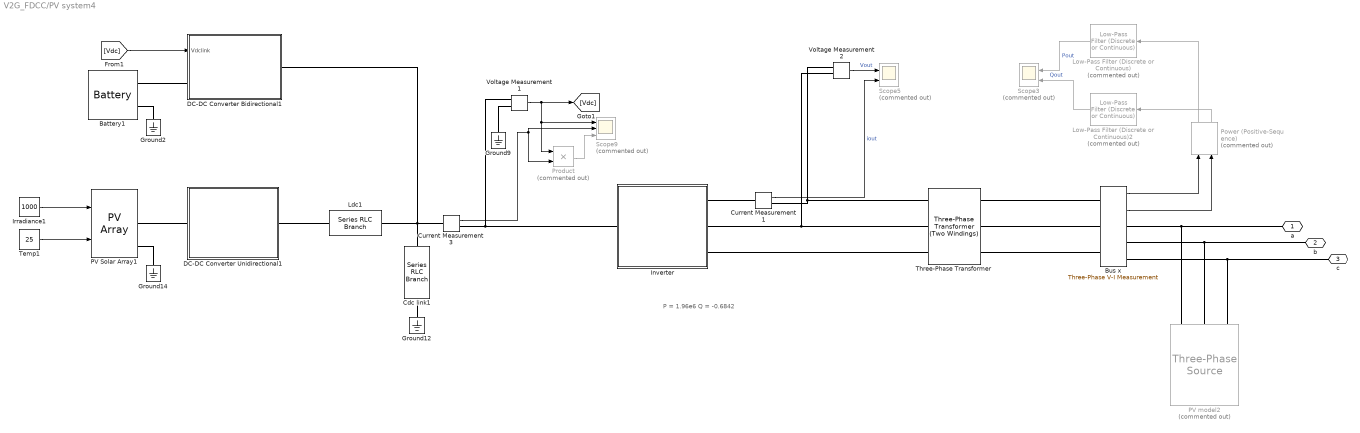
== system V2G_FDCC/PV system4 ==
  note: P = 1.96e6
      | Q = -0.6842
  Battery1 : spsBatteryLib/Battery  BatType=Lead-Acid  ShowTempParam=off  ThermalPreset="12.8V  40Ah  (LiFeMgPO4)"  ShowAgeParam=off  NomV=Vbat  NomQ=cap_bat  SOC=50  Batt_Tr=2  PresetModel=off  MaxQ=cap_bat  MinV=0.8*Vbat  FullV=1.1*Vbat  Dis_rate=Inom_bat  R=0.002  Normal_OP=0.9*cap_bat  expZone="[780   20]"  current=[250 500 750 1000]  Units=Ampere-hour  Tci=20  NomT=20  T2=-30  MaxQ2=4.8  FullV2=7.1  Normal_OP2=5.655  expZone2="[6.58           1]"  Rca=0.6  ti=2000  Dp=0  Neq0=0  Tsim=1e6  Ta1=25  Qeol=5.4*0.9  Reol=0.013333*1.2  Char_age=[2.3478, 3]  Dis_age=[2.3478, 10]  N1=1500  N2=10500  N3=1000  N4=1400  Ta2=45  N5=950
  Bus x : spsThreePhaseVIMeasurementLib/Three-Phase V-I Measurement  VoltageMeasurement=phase-to-ground  SetLabelV=off  LabelV=Vabc  Vpu=off  VpuLL=off  CurrentMeasurement=yes  SetLabelI=off  LabelI=Iabc  Ipu=off  Pbase=100e6  Vbase=13.8e3  OutputType=Complex  PhasorSimulation=off  PSBequivalent=0
  Cdc link1 : spsSeriesRLCBranchLib/Series RLC Branch  LConnTagsString=__new0  RConnTagsString=__new0  BranchType=C  Resistance=0.001  Inductance=1e-3  SetiL0=off  InitialCurrent=0  Capacitance=Cdc  Setx0=on  InitialVoltage=1500  Measurements=None
  Current Measurement1 : spsCurrentMeasurementLib/Current Measurement  PhasorSimulation=off  OutputType=Complex  PSBequivalent=0
  Current Measurement3 : spsCurrentMeasurementLib/Current Measurement  PhasorSimulation=off  OutputType=Complex  PSBequivalent=0
  DC-DC Converter Bidirectional1 : Subsystem
  DC-DC Converter Unidirectional1 : Subsystem
  Ground{2,9,12,14} (4 alike) : spsGroundLib/Ground  LConnTagsString=a
  Inverter : Subsystem
  Irradiance1 : Constant  Value=1000
  Ldc1 : spsSeriesRLCBranchLib/Series RLC Branch  LConnTagsString=__new0  RConnTagsString=__new0  BranchType=L  Resistance=0.002  Inductance=10e-3  SetiL0=off  InitialCurrent=0  Capacitance=5e-3  Setx0=on  InitialVoltage=0  Measurements=None
  Low-Pass Filter (Discrete or Continuous) : eeGeneralControl/Low-Pass Filter (Discrete or Continuous)  Commented=on  K=1  T=1/(2*pi*5)  B=inf  A=-inf  init_option=Inherited from block input  x0=0  Ts=-1
  Low-Pass Filter (Discrete or Continuous)2 : eeGeneralControl/Low-Pass Filter (Discrete or Continuous)  Commented=on  K=1  T=1/(2*pi*5)  B=inf  A=-inf  init_option=Inherited from block input  x0=0  Ts=-1
  PV Solar Array1 : spsPVArrayLib/PV Array  Npar=278  Nser=15  PlotType=array @ 1000 W/m2 & specified temperatures  S_vec=[ 1000 800 500 300 100 ]  Temp_C_vec=[ 20 25 30 35 ]  ModuleName=Sunpower SPR-X22-480-COM  PlotWhenSelected=off  Pm=480.32  Ncell=128  Voc=92.9  Isc=6.48  Vm=79  Im=6.08  beta_Voc_pc=-0.293  alpha_Isc_pc=0.031003  beta_Voc=-0.2722  alpha_Isc=0.002009  IL=6.4884  I0=1.5908e-11  nI=1.0576  Rsh=598.2816  Rs=0.48607  RobustModel=off  RobustCellTemperature=313.3991  BAL=on  Tc=1e-6  Tfilter=5e-5
  PV model2 : spsThreePhaseSourceLib/Three-Phase Source  Commented=on  InternalConnection=Yg  VoltagePhases=off  Voltage=(345000)*1  PhaseAngle=0  Voltage_phases=[25e3 25e3 25e3]/sqrt(3)  PhaseAngles_phases=[0 -120 +120]  Frequency=fg  NonIdealSource=off  SpecifyImpedance=off  Resistance=0.8929  Inductance=16.58e-3  ShortCircuitLevel=100e6  BaseVoltage=25e3  XRratio=7  BusType=swing  Pref=1993000  Qref=10680  Prefabc=[10e3, 10e3, 10e3]  Qrefabc=[0, 0, 0]  Qmin=-Inf  Qmax=Inf
  Power (Positive-Sequence) : spsPowerPositiveSequenceLib/Power (Positive-Sequence)  Commented=on  Freq=50  Vinit=[0, 0]  Iinit=[0, 0]  Ts=1e-5
      settings: LibrarySourceBlock=|
      | sps_lib/Sensors and Measurements/Power
      | (Positive-Sequence)
  Product : Product  Commented=on
  Scope3 : Scope  Commented=on  NumInputPorts=2
  Scope5 : Scope  Commented=on  NumInputPorts=2
  Scope9 : Scope  Commented=on  NumInputPorts=3
  Temp1 : Constant  Value=25
  Three-Phase Transformer : spsThreePhaseTransformerTwoWindingsLib/Three-Phase Transformer (Two Windings)  Winding1Connection=Yg  Winding2Connection=Delta (D1)  CoreType=Three single-phase transformers  SetSaturation=off  Hysteresis=off  DataFile='hysteresis'  SetInitialFlux=off  Measurements=None  UNITS=pu  NominalPower=[ Pinv*2 , fg ]  Winding1=[Vbase 1e-6 1e-6]  Winding2=[Vac_inv 1e-6 1e-6]  Rm=500  Lm=1000  L0=0.5  Saturation=[0 0;0.01 0.9;0.05 1]  InitialFluxes=[-1.0025142026259 0.501432695325379 0.501081507300505]  BreakLoop=off  DiscreteSolver=Trapezoidal iterative  DataType=off  TransfoNumber=1
  Voltage Measurement1 : spsVoltageMeasurementLib/Voltage Measurement  PhasorSimulation=off  OutputType=Complex  PSBequivalent=0
  Voltage Measurement2 : spsVoltageMeasurementLib/Voltage Measurement  PhasorSimulation=off  OutputType=Complex  PSBequivalent=0
  a : PMIOPort  Side=Right
  b : PMIOPort  Port=2  Side=Right
  c : PMIOPort  Port=3  Side=Right
  wires:
  Voltage Measurement2/1 -> Scope5/1  "Vout"
  Irradiance1/1 -> PV Solar Array1/1
  Low-Pass Filter (Discrete or Continuous)/1 -> Scope3/1  "Pout"
  Power (Positive-Sequence)/1 -> Low-Pass Filter (Discrete or Continuous)/1
  Current Measurement1/1 -> Scope5/2  "iout"
  Voltage Measurement1/1 -> [Vdc], Product/1, Scope9/1
  Current Measurement3/1 -> Product/2, Scope9/2
  Low-Pass Filter (Discrete or Continuous)2/1 -> Scope3/2  "Qout"
  [Vdc] -> DC-DC Converter Bidirectional1/1(Vdclink)
  Bus x/2 -> Power (Positive-Sequence)/2
  Temp1/1 -> PV Solar Array1/2
  Bus x/1 -> Power (Positive-Sequence)/1
  Power (Positive-Sequence)/2 -> Low-Pass Filter (Discrete or Continuous)2/1
  Product/1 -> Scope9/3
  connections:
  Inverter/RConn1 -- Current Measurement1/LConn1
  PV Solar Array1/RConn1 -- DC-DC Converter Unidirectional1/LConn1
  Voltage Measurement2/LConn1 -- Current Measurement1/RConn1 -- Three-Phase Transformer/RConn1
  Voltage Measurement2/LConn2 -- Inverter/RConn2 -- Three-Phase Transformer/RConn2
  Inverter/LConn1 -- Voltage Measurement1/LConn1 -- Current Measurement3/RConn1
  Three-Phase Transformer/RConn3 -- Inverter/RConn3
  Battery1/LConn2 -- Ground2/LConn1
  Three-Phase Transformer/LConn3 -- Bus x/LConn3
  Voltage Measurement1/LConn2 -- Ground9/LConn1
  PV Solar Array1/RConn2 -- Ground14/LConn1
  Battery1/LConn1 -- DC-DC Converter Bidirectional1/LConn1
  Ground12/LConn1 -- Cdc link1/RConn1
  Three-Phase Transformer/LConn1 -- Bus x/LConn1
  Current Measurement3/LConn1 -- Cdc link1/LConn1 -- DC-DC Converter Bidirectional1/RConn1 -- Ldc1/RConn1
  Three-Phase Transformer/LConn2 -- Bus x/LConn2
  Ldc1/LConn1 -- DC-DC Converter Unidirectional1/RConn1
  Bus x/RConn2 -- b/RConn1 -- PV model2/RConn2
  Bus x/RConn1 -- a/RConn1 -- PV model2/RConn1
  Bus x/RConn3 -- c/RConn1 -- PV model2/RConn3
